simulink subsystem "Autonomously_Navigate_Poses"  (R2023b)
settings: Solver=VariableStepAuto  StartTime=0.0  StopTime=10.0  RelTol=1e-3
undefined symbols (not defined in the file): Spline_Max_Num_RefPoses, Spline_Num_Samples
settings Model: Creator=FIRSTMentor  LastModifiedBy=ander

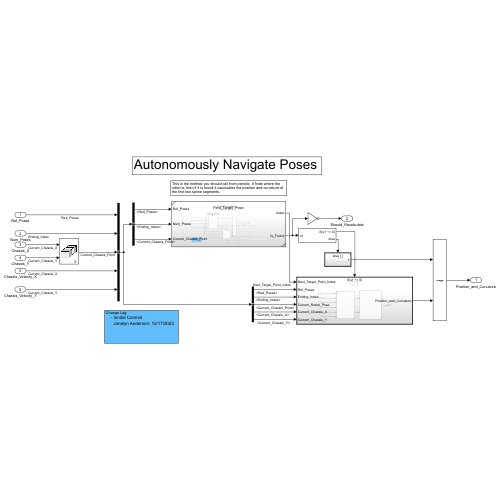
[thumbnail: Simulink's stored preview of the top-level diagram]
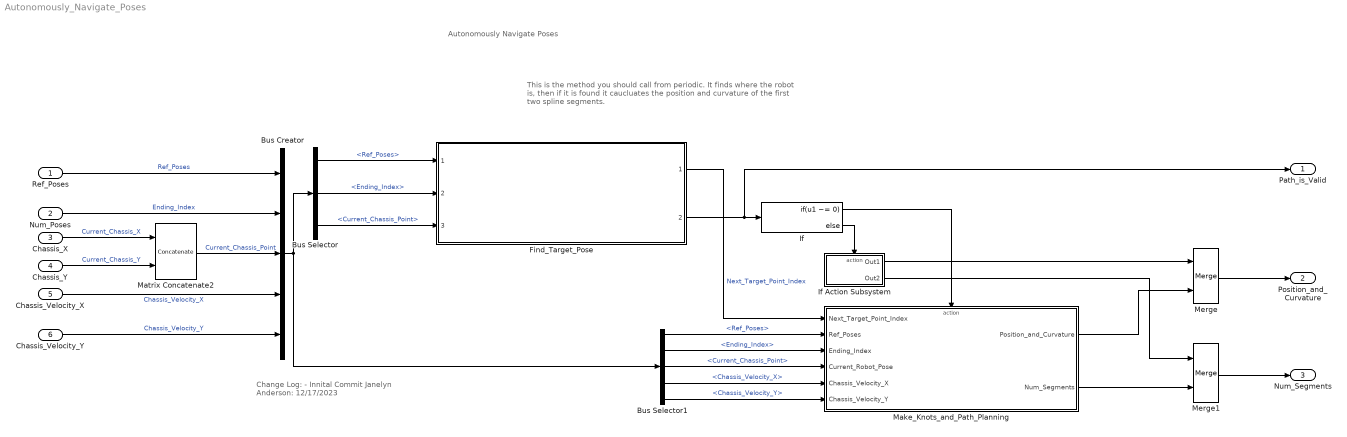
== system Autonomously_Navigate_Poses ==
  note: Autonomously Navigate Poses
  note: This is the method you should call from periodic. It finds where the robot is, then if it is found it caucluates the position and curvature of the first two spline segments.
  note: Change Log:
      | - Innital Commit
      | Janelyn Anderson: 12/17/2023
  Ref_Poses : Inport  OutDataTypeStr=double  PortDimensions=[Spline_Max_Num_RefPoses 2]
  Num_Poses : Inport  Port=2  OutDataTypeStr=int32  Unit=1  PortDimensions=1
  Chassis_X : Inport  Port=3  OutDataTypeStr=double  Unit=m  PortDimensions=1
  Chassis_Y : Inport  Port=4  OutDataTypeStr=double  Unit=m  PortDimensions=1
  Chassis_Velocity_X : Inport  Port=5  OutDataTypeStr=double  Unit=m  PortDimensions=1
  Chassis_Velocity_Y : Inport  Port=6  OutDataTypeStr=double  Unit=m  PortDimensions=1
  Bus Creator : BusCreator  Inputs=5
  Bus Selector : BusSelector  OutputSignals=Ref_Poses,Ending_Index,Current_Chassis_Point
  Bus Selector1 : BusSelector  OutputSignals=Ref_Poses,Ending_Index,Current_Chassis_Point,Chassis_Velocity_X,Chassis_Velocity_Y
  Find_Target_Pose : Subsystem  ReferencedSubsystem=Find_Target_Pose
  If : If  IfExpression=u1 ~= 0
  If Action Subsystem : Subsystem  TreatAsAtomicUnit=on
  Make_Knots_and_Path_Planning : Subsystem
  Matrix Concatenate2 : Concatenate  Mode=Multidimensional array  ConcatenateDimension=2
  Merge : Merge
  Merge1 : Merge
  Path_is_Valid : Outport
  Position_and_Curvature : Outport  Port=2  PortDimensions=[Spline_Num_Samples,3,2]
  Num_Segments : Outport  Port=3
  wires:
  If/2 -> If Action Subsystem/Action
  Bus Selector1/3 -> Make_Knots_and_Path_Planning/4(Current_Robot_Pose)  "<Current_Chassis_Point>"
  Bus Selector1/5 -> Make_Knots_and_Path_Planning/6(Chassis_Velocity_Y)  "<Chassis_Velocity_Y>"
  Find_Target_Pose/2 -> If/1, Path_is_Valid/1
  Merge/1 -> Position_and_Curvature/1
  If Action Subsystem/1(Out1) -> Merge/1
  Bus Selector1/1 -> Make_Knots_and_Path_Planning/2(Ref_Poses)  "<Ref_Poses>"
  Bus Selector/3 -> Find_Target_Pose/3  "<Current_Chassis_Point>"
  Bus Selector1/2 -> Make_Knots_and_Path_Planning/3(Ending_Index)  "<Ending_Index>"
  Bus Creator/1 -> Bus Selector1/1, Bus Selector/1
  Bus Selector1/4 -> Make_Knots_and_Path_Planning/5(Chassis_Velocity_X)  "<Chassis_Velocity_X>"
  If/1 -> Make_Knots_and_Path_Planning/Action
  Bus Selector/1 -> Find_Target_Pose/1  "<Ref_Poses>"
  Num_Poses/1 -> Bus Creator/2  "Ending_Index"
  Bus Selector/2 -> Find_Target_Pose/2  "<Ending_Index>"
  Make_Knots_and_Path_Planning/1(Position_and_Curvature) -> Merge/2
  Chassis_Velocity_X/1 -> Bus Creator/4  "Chassis_Velocity_X"
  Find_Target_Pose/1 -> Make_Knots_and_Path_Planning/1(Next_Target_Point_Index)  "Next_Target_Point_Index"
  Chassis_Velocity_Y/1 -> Bus Creator/5  "Chassis_Velocity_Y"
  Ref_Poses/1 -> Bus Creator/1  "Ref_Poses"
  Matrix Concatenate2/1 -> Bus Creator/3  "Current_Chassis_Point"
  Chassis_Y/1 -> Matrix Concatenate2/2  "Current_Chassis_Y"
  Chassis_X/1 -> Matrix Concatenate2/1  "Current_Chassis_X"
  Make_Knots_and_Path_Planning/2(Num_Segments) -> Merge1/2
  Merge1/1 -> Num_Segments/1
  If Action Subsystem/2(Out2) -> Merge1/1

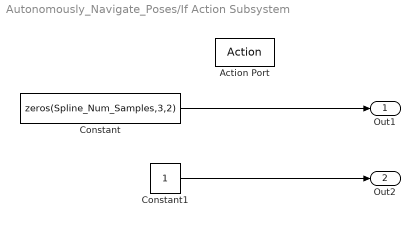
== system Autonomously_Navigate_Poses/If Action Subsystem ==
  Action Port : ActionPort
  Constant : Constant  Value=zeros(Spline_Num_Samples,3,2)
  Constant1 : Constant  OutDataTypeStr=int32
  Out1 : Outport
  Out2 : Outport  Port=2
  wires:
  Constant1/1 -> Out2/1
  Constant/1 -> Out1/1

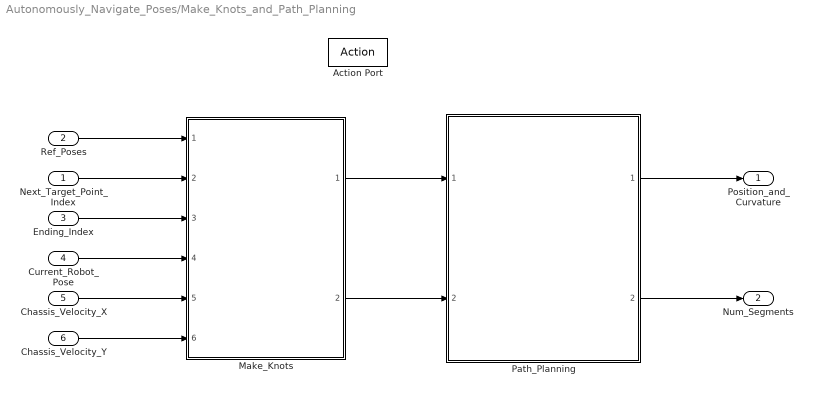
== system Autonomously_Navigate_Poses/Make_Knots_and_Path_Planning ==
  Next_Target_Point_Index : Inport
  Ref_Poses : Inport  Port=2
  Ending_Index : Inport  Port=3
  Current_Robot_Pose : Inport  Port=4
  Chassis_Velocity_X : Inport  Port=5
  Chassis_Velocity_Y : Inport  Port=6
  Action Port : ActionPort  PropagateVarSize=During execution
  Make_Knots : Subsystem  ReferencedSubsystem=Make_Knots
  Path_Planning : Subsystem  ReferencedSubsystem=Path_Planning
  Position_and_Curvature : Outport  PortDimensions=[Spline_Num_Samples,3,2]
  Num_Segments : Outport  Port=2
  wires:
  Path_Planning/2 -> Num_Segments/1
  Chassis_Velocity_Y/1 -> Make_Knots/6
  Current_Robot_Pose/1 -> Make_Knots/4
  Ref_Poses/1 -> Make_Knots/1
  Chassis_Velocity_X/1 -> Make_Knots/5
  Next_Target_Point_Index/1 -> Make_Knots/2
  Ending_Index/1 -> Make_Knots/3
  Make_Knots/1 -> Path_Planning/1
  Make_Knots/2 -> Path_Planning/2
  Path_Planning/1 -> Position_and_Curvature/1
